simulink model "project1"  (R2018b)
settings: Solver=VariableStepAuto  StartTime=0.0  StopTime=10.0  RelTol=1e-3
values from neighbouring files (symbols this model uses):
  A = [0 1; -1 0]    [progetto1.m]    (also in progetto1_modificato.m; progetto_principale1.m; prova1.m)
  Ad = sysd.A    [progetto1.m]    (also in progetto1_modificato.m; progetto_principale1.m; prova1.m)
  B = [0 1]'    [progetto1.m]    (also in progetto1_modificato.m; progetto_principale1.m; prova1.m)
  Bd = sysd.B    [progetto1.m]    (also in progetto1_modificato.m; progetto_principale1.m; prova1.m)
  C = [0 1 ... (first row only)    [progetto1.m]    (also in progetto1_modificato.m; progetto_principale1.m; prova1.m = eye(2))
  D = 0    [progetto1.m]    (also in progetto1_modificato.m; progetto_principale1.m; prova1.m = [0 0]')
  K = [k(:,:,t+1) zeros(2,1) ... (first row only)    [progetto1_modificato.m]
  x0 = [0 1]'    [progetto1.m]    (also in progetto1_modificato.m; progetto_principale1.m; prova1.m)
undefined symbols (not defined in the file or in its folder): Discrete, Time
libraries: simulink x3, ctrlSharedLib x1
settings Model: Creator=Cheng  LastModifiedBy=Cheng

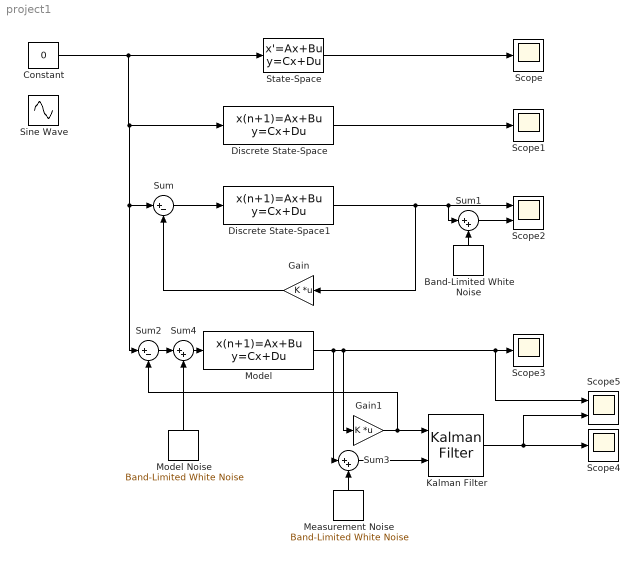
== system project1 ==
  Band-Limited White Noise : simulink/Sources/Band-Limited White Noise  Cov=[0.0001]  Ts=0.1  seed=[23341]
  Constant : Constant  Value=0
  Discrete State-Space : DiscreteStateSpace  A=Ad  B=Bd  C=C  D=D  InitialCondition=x0  SampleTime=-1
  Discrete State-Space1 : DiscreteStateSpace  A=Ad  B=Bd  C=C  D=D  InitialCondition=x0  SampleTime=-1
  Gain : Gain  Gain=K  Multiplication=Matrix(K*u) (u vector)
  Gain1 : Gain  Gain=K  Multiplication=Matrix(K*u) (u vector)
  Kalman Filter : ctrlSharedLib/Kalman Filter  TimeDomain=Discrete-Time  UseCurrentEstimator=on  ModelSource=LTI State-Space Variable  ModelSourceVariable=sysd  A=0.95  B=1  C=1  D=0  NumberOfStates=1  NumberOfInputs=1  NumberOfOutputs=1  InitialEstimateSource=Dialog  X0=x0  P0=10  UseK=off  UseGH=off  NumberOfProcessNoiseInputs=1  G=1  TimeInvariantG=on  H=0  TimeInvariantH=on  Q=0.05  TimeInvariantQ=on  R=1  TimeInvariantR=on  N=0  TimeInvariantN=on  AddInputPort=on  AddEnablePort=off  OutputEstimatedY=off  OutputP=off  Ts=-1
      settings: SourceProductBaseCode=CT
  Measurement Noise : simulink/Sources/Band-Limited White Noise  Cov=[0.0001]  Ts=0.1  seed=[23341]
  Model : DiscreteStateSpace  A=Ad  B=Bd  C=C  D=D  InitialCondition=x0  SampleTime=-1
  Model Noise : simulink/Sources/Band-Limited White Noise  Cov=[0.0001]  Ts=0.1  seed=[23341]
  Scope{,1,3..4} (4 alike) : Scope
  Scope2 : Scope  NumInputPorts=2
  Scope5 : Scope  NumInputPorts=2
  Sine Wave : Sin  Amplitude=4  Frequency=2  Phase=10  SampleTime=0
  State-Space : StateSpace  A=A  B=B  C=C  D=D  InitialCondition=x0
  Sum : Sum  Inputs=|+-
  Sum1 : Sum  Inputs=|++
  Sum2 : Sum  Inputs=|+-
  Sum3 : Sum  Inputs=|++
  Sum4 : Sum  Inputs=|++
  wires:
  State-Space/1 -> Scope/1
  Constant/1 -> Sum2/1, Sum/1, Discrete State-Space/1, State-Space/1
  Discrete State-Space/1 -> Scope1/1
  Discrete State-Space1/1 -> Gain/1, Sum1/1, Scope2/1
  Gain/1 -> Sum/2
  Sum/1 -> Discrete State-Space1/1
  Gain1/1 -> Kalman Filter/1, Sum2/2
  Band-Limited White Noise/1 -> Sum1/2
  Sum1/1 -> Scope2/2
  Kalman Filter/1 -> Scope5/2, Scope4/1
  Sum2/1 -> Sum4/1
  Model/1 -> Sum3/1, Scope5/1, Scope3/1, Gain1/1
  Sum3/1 -> Kalman Filter/2
  Measurement Noise/1 -> Sum3/2
  Sum4/1 -> Model/1
  Model Noise/1 -> Sum4/2
